simulink model "Sound_Source"  (R2020a)
settings: Solver=VariableStepAuto  StartTime=0.0  StopTime=10.0  RelTol=1e-3
libraries: dsparch4 x1
settings Model: Creator=dinhm  LastModifiedBy=dinhm

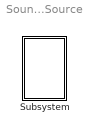
== system Sound_Source ==
  Subsystem : Subsystem

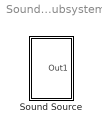
== system Sound_Source/Subsystem ==
  Sound Source : Subsystem

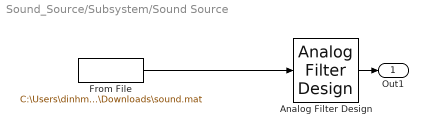
== system Sound_Source/Subsystem/Sound Source ==
  Analog Filter Design : dsparch4/Analog Filter Design  method=Butterworth  filttype=Lowpass  N=8  Wlo=2*pi*4e3  Whi=80  Rp=2  Rs=40
  From File : FromFile  FileName=C:\Users\dinhm\Downloads\sound.mat  SampleTime=0
  Out1 : Outport
  wires:
  From File/1 -> Analog Filter Design/1
  Analog Filter Design/1 -> Out1/1
